simulink model "Folding_QPSK_Costas_modifcations"  (R2019a)
settings: Solver=VariableStepAuto  StartTime=0.0  StopTime=10.0  RelTol=1e-3
libraries: simulink x1, commrandsrc3 x1, commutil2 x1, rfmathmodels1 x1, commdigbbndam3 x1
settings Model: Creator=dom  LastModifiedBy=dom

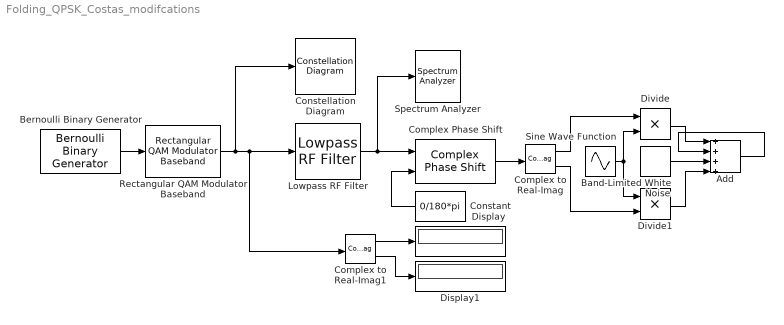
== system Folding_QPSK_Costas_modifcations ==
  Add : Sum  Inputs=++++
  Band-Limited White Noise : simulink/Sources/Band-Limited White Noise  Cov=[0.00000001]  Ts=1e-8  seed=[23341]
  Bernoulli Binary Generator : commrandsrc3/Bernoulli Binary Generator  ProbabilityOfZero=0.5  SeedSource=Parameter  Seed=37  SampleTime=2e-6  SamplesPerFrame=1  OutputDataType=double  SimulateUsing=Interpreted execution
      settings: SourceProductName=Communications Toolbox
  Complex Phase Shift : commutil2/Complex Phase Shift
      settings: SourceProductName=Communications Toolbox  SourceProductBaseCode=CM
  Complex to Real-Imag : ComplexToRealImag
  Complex to Real-Imag1 : ComplexToRealImag
  Constant : Constant  Value=0/180*pi
  Constellation Diagram : ConstellationDiagram
  Display : Display
  Display1 : Display
  Divide : Product  Inputs=**
  Divide1 : Product  Inputs=**
  Lowpass RF Filter : rfmathmodels1/Lowpass RF Filter  method=Butterworth  filttype=Lowpass  N=3  flo=1.9998e6  fhi=2.0002e9  Rp=1  Rs=10  MaxLength=32  Fc=2e6  Ts=2e-6
      settings: SourceProductName=RF Blockset  SourceProductBaseCode=RB
  Rectangular QAM Modulator Baseband : commdigbbndam3/Rectangular QAM Modulator Baseband  M=4  InType=Integer  Enc=Gray  Mapping=[0:15]  PowType=Min. distance between symbols  MinDist=2  AvgPow=1  PeakPow=1  Ph=0  outDtype=double  outWordLen=16  outUDDataType=sfix(16)  outFracLenMode=Best precision  outFracLen=15  outDataTypeStr=double  outLastDataTypeStr=double
      settings: SourceProductName=Communications Toolbox
  Sine Wave Function : Sin  Frequency=2*pi*5e6  SampleTime=1e8
  Spectrum Analyzer : SpectrumAnalyzer
  wires:
  Rectangular QAM Modulator Baseband/1 -> Constellation Diagram/1, Lowpass RF Filter/1, Complex to Real-Imag1/1
  Constant/1 -> Complex Phase Shift/2
  Complex to Real-Imag1/1 -> Display/1
  Complex to Real-Imag1/2 -> Display1/1
  Complex Phase Shift/1 -> Complex to Real-Imag/1
  Divide/1 -> Add/1
  Bernoulli Binary Generator/1 -> Rectangular QAM Modulator Baseband/1
  Lowpass RF Filter/1 -> Spectrum Analyzer/1, Complex Phase Shift/1
  Divide1/1 -> Add/4
  Band-Limited White Noise/1 -> Add/3
  Sine Wave Function/1 -> Divide1/1, Divide/2
  Complex to Real-Imag/1 -> Divide/1
  Complex to Real-Imag/2 -> Divide1/2
  Add/1 -> Add/2
